simulink model "Motors_PID_Simulink_Main"  (R2019b)
settings: Solver=VariableStepAuto  StartTime=0.0  StopTime=10  FixedStep=0.0001  RelTol=1e-3
values from neighbouring files (symbols this model uses):
  desired_angle_vectors = [pi/2 -1.57 1.57/2 -pi/4]    [Motors_Main_Project.m]
  EB = B(3)    [Motors_Main_Project.m]
  EJ = J(3)    [Motors_Main_Project.m]
  EKb = Kb(3)    [Motors_Main_Project.m]
  EKm = Km(3)    [Motors_Main_Project.m]
  EL = L(3)    [Motors_Main_Project.m]
  res = (2*pi)/CPR    (= 0.0490873852123)    [Motors_Main_Project.m]
  SB = B(4)    [Motors_Main_Project.m]
  SJ = J(4)    [Motors_Main_Project.m]
  SKb = Kb(4)    [Motors_Main_Project.m]
  SKm = Km(4)    [Motors_Main_Project.m]
  SL = L(4)    [Motors_Main_Project.m]
  WB = B(2)    [Motors_Main_Project.m]
  WJ = J(2)    [Motors_Main_Project.m]
  WKb = Kb(2)    [Motors_Main_Project.m]
  WKm = Km(2)    [Motors_Main_Project.m]
  WL = L(2)    [Motors_Main_Project.m]
undefined symbols (not defined in the file or in its folder): ER, GR, SR
libraries: cstblocks x4, simulink x4
settings Model: Creator=harsh  LastModifiedBy=harsh

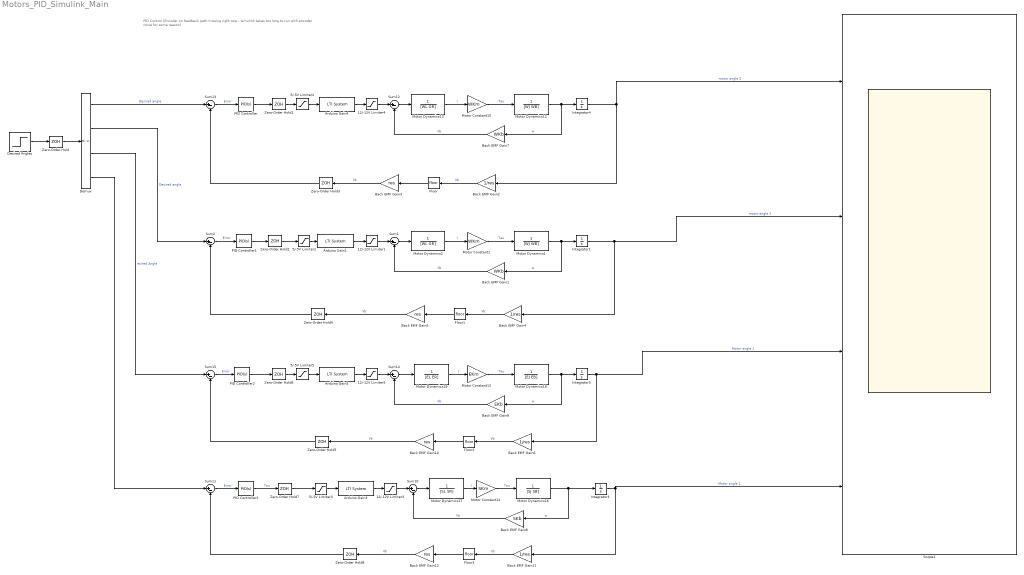
== system Motors_PID_Simulink_Main ==
  note: PID Control
      | (Encoder on feedback path missing right now - simulink takes too long to run with encoder noise for some reason)
  12/-12V Limiter{1,3..5} (4 alike) : Saturate  UpperLimit=12  LowerLimit=-12
  5/-5V Limiter{1,3..5} (4 alike) : Saturate  UpperLimit=5  LowerLimit=-5
  Arduino Gain1 : cstblocks/LTI System  sys=WOPAMP  IC=[]
  Arduino Gain3 : cstblocks/LTI System  sys=SOPAMP  IC=[]
  Arduino Gain4 : cstblocks/LTI System  sys=GOPAMP  IC=[]
  Arduino Gain5 : cstblocks/LTI System  sys=EOPAMP  IC=[]
  Back EMF Gain1 : Gain  Gain=WKb
  Back EMF Gain{3,5,10,12} (4 alike) : Gain  Gain=res
  Back EMF Gain{2,4,6,11} (4 alike) : Gain  Gain=1/res
  Back EMF Gain7 : Gain  Gain=WKb
  Back EMF Gain8 : Gain  Gain=SKb
  Back EMF Gain9 : Gain  Gain=EKb
  Demux : Demux
  "Desired Angles " : Step  After=desired_angle_vectors  SampleTime=0
  Floor{,1..3} (4 alike) : Rounding
  Integrator{1,3..5} (4 alike) : Integrator
  Motor Constant1 : Gain  Gain=WKm
  Motor Constant10 : Gain  Gain=WKm
  Motor Constant12 : Gain  Gain=SKm
  Motor Constant13 : Gain  Gain=EKm
  Motor Dynamics1 : TransferFcn  Denominator=[WJ WB]
  Motor Dynamics12 : TransferFcn  Denominator=[WJ WB]
  Motor Dynamics13 : TransferFcn  Denominator=[WL GR]
  Motor Dynamics16 : TransferFcn  Denominator=[SJ SB]
  Motor Dynamics17 : TransferFcn  Denominator=[SL SR]
  Motor Dynamics18 : TransferFcn  Denominator=[EJ EB]
  Motor Dynamics19 : TransferFcn  Denominator=[EL ER]
  Motor Dynamics2 : TransferFcn  Denominator=[WL GR]
  PID Controller : simulink/Continuous/PID Controller  Controller=PID  Form=Parallel  TimeDomain=Continuous-time  SampleTime=-1  IntegratorMethod=Forward Euler  FilterMethod=Forward Euler  ControllerParametersSource=internal  P=7.3697  I=24.525  D=0.04744  UseFilter=on  N=5000  TunerSelectOption=Transfer Function Based (PID Tuner App)  InitialConditionSource=internal  InitialConditionForIntegrator=0  InitialConditionForFilter=0  DifferentiatorICPrevScaledInput=0  ExternalReset=none  TrackingMode=off  Kt=1  LimitOutput=off  UpperSaturationLimit=inf  LowerSaturationLimit=-inf  LinearizeAsGain=on  AntiWindupMode=none  Kb=1  POutMin=[]  POutMax=[]  IOutMin=[]  IOutMax=[]  DOutMin=[]  DOutMax=[]  NOutMin=[]  NOutMax=[]  SumOutMin=[]  SumOutMax=[]  SaturationOutMin=[]  SaturationOutMax=[]  PParamMin=[]  PParamMax=[]  IParamMin=[]  IParamMax=[]  DParamMin=[]  DParamMax=[]  NParamMin=[]  NParamMax=[]  KbParamMin=[]  KbParamMax=[]  KtParamMin=[]  KtParamMax=[]  KbOutMin=[]  KbOutMax=[]  KtOutMin=[]  KtOutMax=[]  IntegratorOutMin=[]  IntegratorOutMax=[]  FilterOutMin=[]  FilterOutMax=[]  SumI1OutMin=[]  SumI1OutMax=[]  SumI2OutMin=[]  SumI2OutMax=[]  SumI3OutMin=[]  SumI3OutMax=[]  SumI4OutMin=[]  SumI4OutMax=[]  SumDOutMin=[]  SumDOutMax=[]  DifferentiatorOutMin=[]  DifferentiatorOutMax=[]  FilterDiffOutCoefMin=[]  FilterDiffOutCoefMax=[]  ReciprocalOutMin=[]  ReciprocalOutMax=[]  SumDenOutMin=[]  SumDenOutMax=[]  SumNumOutMin=[]  SumNumOutMax=[]  DivideOutMin=[]  DivideOutMax=[]  IntegratorContinuousStateAttributes=''  IntegratorStateMustResolveToSignalObject=off  IntegratorRTWStateStorageClass=Auto  FilterContinuousStateAttributes=''  FilterStateMustResolveToSignalObject=off  FilterRTWStateStorageClass=Auto  ParallelPVariant=InternalParameters  IdealPVariant=Disabled  IVariant=InternalParameters  DVariant=InternalParameters  IntegratorVariant=Continuous  SatVariant=Disabled  AWVariant=Passthrough  PCopyVariant=Disabled  TRVariant=Disabled  FdbkBlocksVariant=Forward  IdealPFdbkVariant=Disabled  SatFdbkVariant=Disabled  DerivativeFilterVariant=ContFilter  NVariant=InternalParameters  NCopyVariant=Disabled  FilterICVariant=InternalICsFilter  IntegratorICVariant=InternalICs  ExternalResetVariant=Disabled  TRSumVariant=Passthrough  SumFdbkVariant=Disabled  SumVariant=Sum_PID
  PID Controller1 : simulink/Continuous/PID Controller  Controller=PID  Form=Parallel  TimeDomain=Continuous-time  SampleTime=-1  IntegratorMethod=Forward Euler  FilterMethod=Forward Euler  ControllerParametersSource=internal  P=7.3697  I=24.525  D=0.04744  UseFilter=on  N=5000  TunerSelectOption=Transfer Function Based (PID Tuner App)  InitialConditionSource=internal  InitialConditionForIntegrator=0  InitialConditionForFilter=0  DifferentiatorICPrevScaledInput=0  ExternalReset=none  TrackingMode=off  Kt=1  LimitOutput=off  UpperSaturationLimit=inf  LowerSaturationLimit=-inf  LinearizeAsGain=on  AntiWindupMode=none  Kb=1  POutMin=[]  POutMax=[]  IOutMin=[]  IOutMax=[]  DOutMin=[]  DOutMax=[]  NOutMin=[]  NOutMax=[]  SumOutMin=[]  SumOutMax=[]  SaturationOutMin=[]  SaturationOutMax=[]  PParamMin=[]  PParamMax=[]  IParamMin=[]  IParamMax=[]  DParamMin=[]  DParamMax=[]  NParamMin=[]  NParamMax=[]  KbParamMin=[]  KbParamMax=[]  KtParamMin=[]  KtParamMax=[]  KbOutMin=[]  KbOutMax=[]  KtOutMin=[]  KtOutMax=[]  IntegratorOutMin=[]  IntegratorOutMax=[]  FilterOutMin=[]  FilterOutMax=[]  SumI1OutMin=[]  SumI1OutMax=[]  SumI2OutMin=[]  SumI2OutMax=[]  SumI3OutMin=[]  SumI3OutMax=[]  SumI4OutMin=[]  SumI4OutMax=[]  SumDOutMin=[]  SumDOutMax=[]  DifferentiatorOutMin=[]  DifferentiatorOutMax=[]  FilterDiffOutCoefMin=[]  FilterDiffOutCoefMax=[]  ReciprocalOutMin=[]  ReciprocalOutMax=[]  SumDenOutMin=[]  SumDenOutMax=[]  SumNumOutMin=[]  SumNumOutMax=[]  DivideOutMin=[]  DivideOutMax=[]  IntegratorContinuousStateAttributes=''  IntegratorStateMustResolveToSignalObject=off  IntegratorRTWStateStorageClass=Auto  FilterContinuousStateAttributes=''  FilterStateMustResolveToSignalObject=off  FilterRTWStateStorageClass=Auto  ParallelPVariant=InternalParameters  IdealPVariant=Disabled  IVariant=InternalParameters  DVariant=InternalParameters  IntegratorVariant=Continuous  SatVariant=Disabled  AWVariant=Passthrough  PCopyVariant=Disabled  TRVariant=Disabled  FdbkBlocksVariant=Forward  IdealPFdbkVariant=Disabled  SatFdbkVariant=Disabled  DerivativeFilterVariant=ContFilter  NVariant=InternalParameters  NCopyVariant=Disabled  FilterICVariant=InternalICsFilter  IntegratorICVariant=InternalICs  ExternalResetVariant=Disabled  TRSumVariant=Passthrough  SumFdbkVariant=Disabled  SumVariant=Sum_PID
  PID Controller2 : simulink/Continuous/PID Controller  Controller=PID  Form=Parallel  TimeDomain=Continuous-time  SampleTime=-1  IntegratorMethod=Forward Euler  FilterMethod=Forward Euler  ControllerParametersSource=internal  P=7.3697  I=10.525  D=0.04744  UseFilter=on  N=5000  TunerSelectOption=Transfer Function Based (PID Tuner App)  InitialConditionSource=internal  InitialConditionForIntegrator=0  InitialConditionForFilter=0  DifferentiatorICPrevScaledInput=0  ExternalReset=none  TrackingMode=off  Kt=1  LimitOutput=off  UpperSaturationLimit=inf  LowerSaturationLimit=-inf  LinearizeAsGain=on  AntiWindupMode=none  Kb=1  POutMin=[]  POutMax=[]  IOutMin=[]  IOutMax=[]  DOutMin=[]  DOutMax=[]  NOutMin=[]  NOutMax=[]  SumOutMin=[]  SumOutMax=[]  SaturationOutMin=[]  SaturationOutMax=[]  PParamMin=[]  PParamMax=[]  IParamMin=[]  IParamMax=[]  DParamMin=[]  DParamMax=[]  NParamMin=[]  NParamMax=[]  KbParamMin=[]  KbParamMax=[]  KtParamMin=[]  KtParamMax=[]  KbOutMin=[]  KbOutMax=[]  KtOutMin=[]  KtOutMax=[]  IntegratorOutMin=[]  IntegratorOutMax=[]  FilterOutMin=[]  FilterOutMax=[]  SumI1OutMin=[]  SumI1OutMax=[]  SumI2OutMin=[]  SumI2OutMax=[]  SumI3OutMin=[]  SumI3OutMax=[]  SumI4OutMin=[]  SumI4OutMax=[]  SumDOutMin=[]  SumDOutMax=[]  DifferentiatorOutMin=[]  DifferentiatorOutMax=[]  FilterDiffOutCoefMin=[]  FilterDiffOutCoefMax=[]  ReciprocalOutMin=[]  ReciprocalOutMax=[]  SumDenOutMin=[]  SumDenOutMax=[]  SumNumOutMin=[]  SumNumOutMax=[]  DivideOutMin=[]  DivideOutMax=[]  IntegratorContinuousStateAttributes=''  IntegratorStateMustResolveToSignalObject=off  IntegratorRTWStateStorageClass=Auto  FilterContinuousStateAttributes=''  FilterStateMustResolveToSignalObject=off  FilterRTWStateStorageClass=Auto  ParallelPVariant=InternalParameters  IdealPVariant=Disabled  IVariant=InternalParameters  DVariant=InternalParameters  IntegratorVariant=Continuous  SatVariant=Disabled  AWVariant=Passthrough  PCopyVariant=Disabled  TRVariant=Disabled  FdbkBlocksVariant=Forward  IdealPFdbkVariant=Disabled  SatFdbkVariant=Disabled  DerivativeFilterVariant=ContFilter  NVariant=InternalParameters  NCopyVariant=Disabled  FilterICVariant=InternalICsFilter  IntegratorICVariant=InternalICs  ExternalResetVariant=Disabled  TRSumVariant=Passthrough  SumFdbkVariant=Disabled  SumVariant=Sum_PID
  PID Controller3 : simulink/Continuous/PID Controller  Controller=PID  Form=Parallel  TimeDomain=Continuous-time  SampleTime=-1  IntegratorMethod=Forward Euler  FilterMethod=Forward Euler  ControllerParametersSource=internal  P=1  I=1  D=1  UseFilter=on  N=100  TunerSelectOption=Transfer Function Based (PID Tuner App)  InitialConditionSource=internal  InitialConditionForIntegrator=0  InitialConditionForFilter=0  DifferentiatorICPrevScaledInput=0  ExternalReset=none  TrackingMode=off  Kt=1  LimitOutput=off  UpperSaturationLimit=inf  LowerSaturationLimit=-inf  LinearizeAsGain=on  AntiWindupMode=none  Kb=1  POutMin=[]  POutMax=[]  IOutMin=[]  IOutMax=[]  DOutMin=[]  DOutMax=[]  NOutMin=[]  NOutMax=[]  SumOutMin=[]  SumOutMax=[]  SaturationOutMin=[]  SaturationOutMax=[]  PParamMin=[]  PParamMax=[]  IParamMin=[]  IParamMax=[]  DParamMin=[]  DParamMax=[]  NParamMin=[]  NParamMax=[]  KbParamMin=[]  KbParamMax=[]  KtParamMin=[]  KtParamMax=[]  KbOutMin=[]  KbOutMax=[]  KtOutMin=[]  KtOutMax=[]  IntegratorOutMin=[]  IntegratorOutMax=[]  FilterOutMin=[]  FilterOutMax=[]  SumI1OutMin=[]  SumI1OutMax=[]  SumI2OutMin=[]  SumI2OutMax=[]  SumI3OutMin=[]  SumI3OutMax=[]  SumI4OutMin=[]  SumI4OutMax=[]  SumDOutMin=[]  SumDOutMax=[]  DifferentiatorOutMin=[]  DifferentiatorOutMax=[]  FilterDiffOutCoefMin=[]  FilterDiffOutCoefMax=[]  ReciprocalOutMin=[]  ReciprocalOutMax=[]  SumDenOutMin=[]  SumDenOutMax=[]  SumNumOutMin=[]  SumNumOutMax=[]  DivideOutMin=[]  DivideOutMax=[]  IntegratorContinuousStateAttributes=''  IntegratorStateMustResolveToSignalObject=off  IntegratorRTWStateStorageClass=Auto  FilterContinuousStateAttributes=''  FilterStateMustResolveToSignalObject=off  FilterRTWStateStorageClass=Auto  ParallelPVariant=InternalParameters  IdealPVariant=Disabled  IVariant=InternalParameters  DVariant=InternalParameters  IntegratorVariant=Continuous  SatVariant=Disabled  AWVariant=Passthrough  PCopyVariant=Disabled  TRVariant=Disabled  FdbkBlocksVariant=Forward  IdealPFdbkVariant=Disabled  SatFdbkVariant=Disabled  DerivativeFilterVariant=ContFilter  NVariant=InternalParameters  NCopyVariant=Disabled  FilterICVariant=InternalICsFilter  IntegratorICVariant=InternalICs  ExternalResetVariant=Disabled  TRSumVariant=Passthrough  SumFdbkVariant=Disabled  SumVariant=Sum_PID
  Scope1 : Scope  NumInputPorts=4
  Sum{1..2,10..15} (8 alike) : Sum  Inputs=|+-
  Zero-Order Hold{,1,3..8} (8 alike) : ZeroOrderHold  SampleTime=0.0001
  Zero-Order Hold2 : ZeroOrderHold  SampleTime=-1
  wires:
  "Desired Angles "/1 -> Zero-Order Hold/1
  5/-5V Limiter4/1 -> Arduino Gain4/1
  Arduino Gain4/1 -> 12/-12V Limiter4/1
  Back EMF Gain7/1 -> Sum12/2  "Vb"
  Sum12/1 -> Motor Dynamics13/1
  Motor Dynamics12/1 -> Back EMF Gain7/1, Integrator4/1  "w"
  Demux/1 -> Sum13/1  "Desired angle"
  12/-12V Limiter4/1 -> Sum12/1
  Motor Dynamics13/1 -> Motor Constant10/1  "I"
  Motor Constant10/1 -> Motor Dynamics12/1  "Tau"
  Sum13/1 -> PID Controller/1  "Error"
  Integrator4/1 -> Scope1/1, Back EMF Gain2/1  "motor angle 2"
  Motor Constant1/1 -> Motor Dynamics1/1  "Tau"
  Sum2/1 -> PID Controller1/1  "Error"
  12/-12V Limiter1/1 -> Sum1/1
  Motor Dynamics2/1 -> Motor Constant1/1  "I"
  Motor Dynamics1/1 -> Back EMF Gain1/1, Integrator1/1  "w"
  Sum1/1 -> Motor Dynamics2/1
  Integrator1/1 -> Scope1/2, Back EMF Gain4/1  "motor angle 2"
  5/-5V Limiter1/1 -> Arduino Gain1/1
  Back EMF Gain1/1 -> Sum1/2  "Vb"
  Arduino Gain1/1 -> 12/-12V Limiter1/1
  Demux/2 -> Sum2/1  "Desired angle"
  PID Controller2/1 -> Zero-Order Hold6/1
  Sum15/1 -> PID Controller2/1  "Error"
  Motor Dynamics19/1 -> Motor Constant13/1  "I"
  Motor Constant13/1 -> Motor Dynamics18/1  "Tau"
  12/-12V Limiter5/1 -> Sum14/1
  Sum14/1 -> Motor Dynamics19/1
  Motor Dynamics18/1 -> Back EMF Gain9/1, Integrator5/1  "w"
  5/-5V Limiter5/1 -> Arduino Gain5/1
  Back EMF Gain9/1 -> Sum14/2  "Vb"
  Arduino Gain5/1 -> 12/-12V Limiter5/1
  Integrator5/1 -> Scope1/3, Back EMF Gain6/1  "Motor angle 1"
  Demux/3 -> Sum15/1  "esired Angle"
  Back EMF Gain8/1 -> Sum10/2  "Vb"
  Motor Constant12/1 -> Motor Dynamics16/1  "Tau"
  Motor Dynamics16/1 -> Back EMF Gain8/1, Integrator3/1  "w"
  5/-5V Limiter3/1 -> Arduino Gain3/1
  Arduino Gain3/1 -> 12/-12V Limiter3/1
  Motor Dynamics17/1 -> Motor Constant12/1  "I"
  12/-12V Limiter3/1 -> Sum10/1
  PID Controller3/1 -> Zero-Order Hold7/1  "Tau"
  Sum11/1 -> PID Controller3/1  "Error"
  Sum10/1 -> Motor Dynamics17/1
  Demux/4 -> Sum11/1
  Integrator3/1 -> Scope1/4, Back EMF Gain11/1  "Motor angle 1"
  PID Controller1/1 -> Zero-Order Hold2/1
  PID Controller/1 -> Zero-Order Hold1/1
  Zero-Order Hold/1 -> Demux/1
  Zero-Order Hold1/1 -> 5/-5V Limiter4/1
  Zero-Order Hold2/1 -> 5/-5V Limiter1/1
  Zero-Order Hold3/1 -> Sum13/2
  Zero-Order Hold4/1 -> Sum2/2
  Zero-Order Hold5/1 -> Sum15/2
  Zero-Order Hold6/1 -> 5/-5V Limiter5/1
  Zero-Order Hold7/1 -> 5/-5V Limiter3/1
  Zero-Order Hold8/1 -> Sum11/2
  Floor/1 -> Back EMF Gain3/1
  Back EMF Gain2/1 -> Floor/1  "Vb"
  Back EMF Gain3/1 -> Zero-Order Hold3/1  "Vb"
  Back EMF Gain4/1 -> Floor1/1  "Vb"
  Back EMF Gain5/1 -> Zero-Order Hold4/1  "Vb"
  Floor1/1 -> Back EMF Gain5/1
  Back EMF Gain6/1 -> Floor2/1  "Vb"
  Floor2/1 -> Back EMF Gain10/1
  Back EMF Gain10/1 -> Zero-Order Hold5/1  "Vb"
  Back EMF Gain11/1 -> Floor3/1  "Vb"
  Floor3/1 -> Back EMF Gain12/1
  Back EMF Gain12/1 -> Zero-Order Hold8/1  "Vb"
